simulink model "Boiler_steam_pressure_control_system"  (R2024a)
settings: Solver=FixedStepAuto  StartTime=0.0  StopTime=3000  FixedStep=0.01  RelTol=1e-3
settings Model: Creator=23204  LastModifiedBy=23204
settings SolverCC: EnableFixedStepZeroCrossing=on
settings OptimizationCC: DefaultParameterBehavior=Inlined  UseDivisionForNetSlopeComputation=on  GainParamInheritBuiltInType=on  UseFloatMulNetSlope=on  InlineInvariantSignals=on  PassReuseOutputArgsAs=Individual arguments  ZeroExternalMemoryAtStartup=off  ZeroInternalMemoryAtStartup=off  NoFixptDivByZeroProtection=on  EfficientFloat2IntCast=on  LifeSpan=1  OptimizeBlockOrder=speed  DifferentSizesBufferReuse=on  EfficientTunableParamExpr=on
settings DebuggingCC: ParameterTunabilityLossMsg=error
settings HardwareCC: ProdLongLongMode=on
settings SFSimCC: MATLABDynamicMemAlloc=off
settings RTWCC: Description=Embedded Coder  SystemTargetFile=ert.tlc  GenCodeOnly=on  TemplateMakefile=ert_default_tmf
settings CodeAppCC: ForceParamTrailComments=on  IgnoreCustomStorageClasses=off  OperatorAnnotations=on  SimulinkDataObjDesc=on  SFDataObjDesc=on  CustomSymbolStrGlobalVar=rt$N$M  CustomSymbolStrType=$N$M  CustomSymbolStrFcn=$N$M$F  CustomSymbolStrMacro=$N$M  InsertBlockDesc=on
settings ERTTargetCC: TargetLangStandard=C99 (ISO)  GenerateSampleERTMain=on  IncludeMdlTerminateFcn=off  CombineSignalStateStructs=on  SupportComplex=off  SupportContinuousTime=on  InlinedParameterPlacement=NonHierarchical  ERTCustomFileTemplate=example_file_process.tlc  ERTFilePackagingFormat=CompactWithDataFile

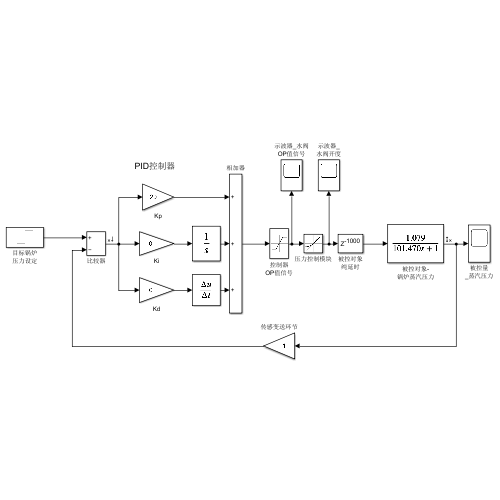
[thumbnail: Simulink's stored preview of the top-level diagram]
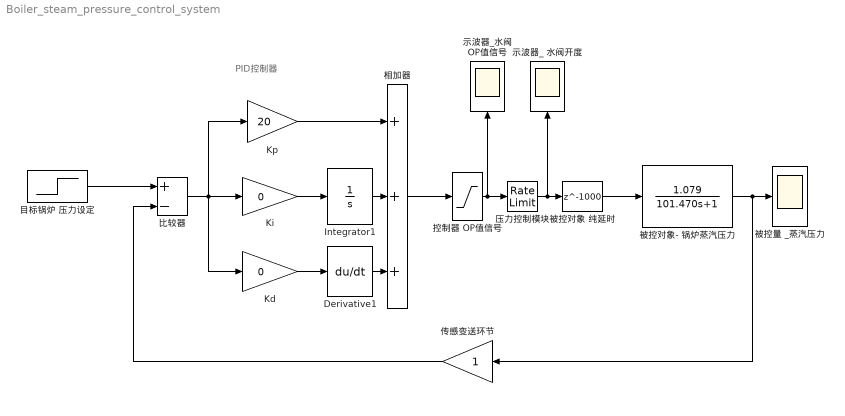
== system Boiler_steam_pressure_control_system ==
  note: PID控制器
  Derivative1 : Derivative
  Integrator1 : Integrator
  Kd : Gain  Gain=0
  Ki : Gain  Gain=0
  Kp : Gain  Gain=20
  传感变送环节 : Gain
  压力控制模块 : RateLimiter  RisingSlewLimit=25  FallingSlewLimit=-25  SampleTimeMode=inherited
  控制器 OP值信号 : Saturate  UpperLimit=99  LowerLimit=1  LinearizeAsGain=off
  比较器 : Sum  Inputs=+-
  "目标锅炉 压力设定 " : Step  After=60  SampleTime=0.01
  相加器 : Sum  Inputs=+++  OutDataTypeStr=double  AccumDataTypeStr=double
  示波器_ 水阀开度 : Scope
  示波器_水阀 OP值信号 : Scope
  被控对象 纯延时 : Delay  DelayLength=1000  SampleTime=0.01
  被控对象- 锅炉蒸汽压力 : TransferFcn  Numerator=[1.079]  Denominator=[101.470 1]
  被控量 _蒸汽压力 : Scope
  wires:
  Kd/1 -> Derivative1/1
  Derivative1/1 -> 相加器/3
  Ki/1 -> Integrator1/1
  比较器/1 -> Kd/1, Kp/1, Ki/1
  Integrator1/1 -> 相加器/2
  Kp/1 -> 相加器/1
  相加器/1 -> 控制器 OP值信号/1
  控制器 OP值信号/1 -> 压力控制模块/1, 示波器_水阀 OP值信号/1
  "目标锅炉 压力设定 "/1 -> 比较器/1
  被控对象- 锅炉蒸汽压力/1 -> 被控量 _蒸汽压力/1, 传感变送环节/1
  压力控制模块/1 -> 示波器_ 水阀开度/1, 被控对象 纯延时/1
  被控对象 纯延时/1 -> 被控对象- 锅炉蒸汽压力/1
  传感变送环节/1 -> 比较器/2
